simulink model "coefficientOfFriction_2017a_directVcommand"  (R2017a)
settings: Solver=FixedStepDiscrete  StartTime=0.0  StopTime=inf  FixedStep=mdl_T_sample  RelTol=1e-3
undefined symbols (not defined in the file): ctrl_angVel_pid_k_d, ctrl_angVel_pid_k_i, ctrl_angVel_pid_k_p, DiscIntNeverNeededParam, gyro_k_raw2rps, gyro_x_bias, gyro_x_reset, gyro_y_bias, gyro_y_reset, gyro_z_bias, gyro_z_reset, io_read_rateTransition_initialCondition, k_intmax_uint8, mdl, mdl_T_sample, mdl_v_supply, mtr_encoder_countPerRev, mtr_encoder_filter_z_den, mtr_encoder_filter_z_num, mtr_encoder_filter_z_ss_A, mtr_encoder_filter_z_ss_B, mtr_encoder_filter_z_ss_C, mtr_encoder_filter_z_ss_D, mtr_encoder_radPerRev, ui_mtr_w_cmd_dmax, ui_mtr_w_cmd_dmin, ui_mtr_w_cmd_rps, ui_mtr_w_cmd_tStart
libraries: svdutilitieslib x14, simulink x6, arduinolib x5, MinSegLibrary_M2V3 x2, RASPlib x1
settings Model: ExtModeTrigDuration=2  Creator=kando  LastModifiedBy=kando
settings DataIOCC: SaveOutput=off  SignalLogging=off  DSMLogging=off  VisualizeSimOutput=off  SaveTime=off
settings OptimizationCC: LifeSpan=Inf  MaxStackSize=64  SimCompilerOptimization=on  AccelVerboseBuild=on
settings DebuggingCC: AllowSymbolicDim=off  SFUnexpectedBacktrackingDiag=warning  SFNoUnconditionalDefaultTransitionDiag=warning  SFExecutionAtInitializationDiag=none
settings HardwareCC: ProdBitPerInt=16  ProdBitPerPointer=16  ProdBitPerSizeT=16  ProdBitPerPtrDiffT=16  ProdLargestAtomicFloat=None  ProdWordSize=8  ProdHWDeviceType=Atmel->AVR  UseEmbeddedCoderFeatures=off  UseSimulinkCoderFeatures=off
settings ModelReferenceCC: PropagateSignalLabelsOutOfModel=off
settings SFSimCC: MATLABDynamicMemAlloc=off
settings RTWCC: SystemTargetFile=ert.tlc  HardwareBoard=Arduino Mega 2560  TLCOptions=-aInlineSetEventsForThisBaseRateFcn=TLC_FALSE -aSuppressMultiTaskScheduler=TLC_FALSE -aRateBasedStepFcn=1  TemplateMakefile=ert_default_tmf  Description=Embedded Coder  Toolchain=Arduino AVR  BuildConfiguration=Faster Runs
settings ERTTargetCC: MultiwordLength=2048  ERTCustomFileBanners=off  SupportContinuousTime=on  SupportNonInlinedSFcns=on  RemoveResetFunc=off  SupportVariableSizeSignals=on  ModelStepFunctionPrototypeControlCompliant=off  ConvertIfToSwitch=off  SuppressUnreachableDefaultCases=off
settings ConfigComp: CovMetricSettings=dw  CovHtmlReporting=on  CovSaveCumulativeToWorkspaceVar=on  CovSaveSingleToWorkspaceVar=on  CovExternalEMLEnable=off

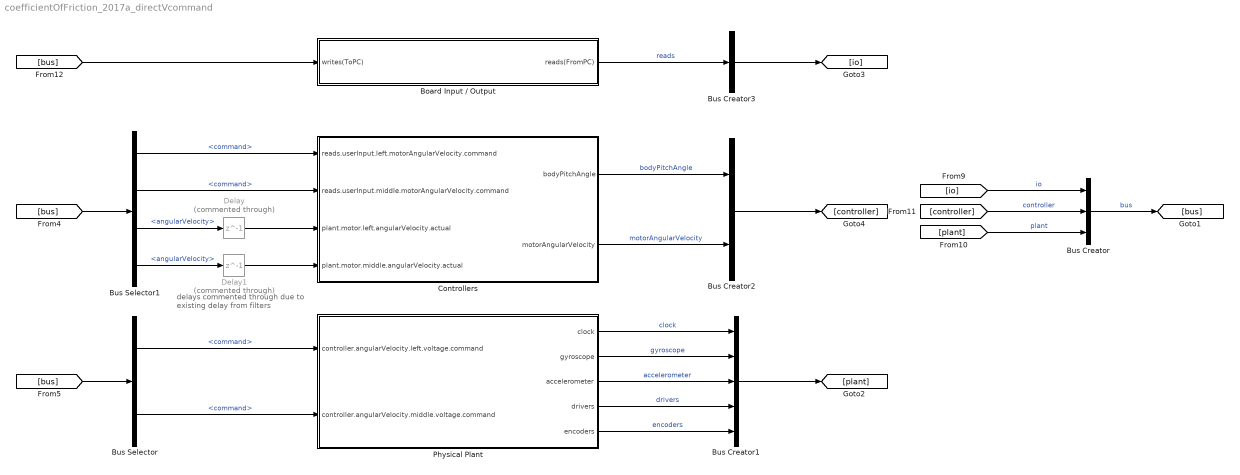
== system coefficientOfFriction_2017a_directVcommand ==
  note: delays commented through
      | due to existing delay from filters
  Board Input / Output : Subsystem
  Bus Creator : BusCreator  Inputs=3
  Bus Creator1 : BusCreator  Inputs=5
  Bus Creator2 : BusCreator  Inputs=2
  Bus Creator3 : BusCreator  Inputs=1
  Bus Selector : BusSelector  OutputSignals=controller.motorAngularVelocity.left.voltage.command,controller.motorAngularVelocity.middle.voltage.command
  Bus Selector1 : BusSelector  OutputSignals=io.reads.userInput.motorAngularVelocity.command,io.reads.userInput.motorAngularVelocity.command,plant.encoders.left.angularVelocity,plant.encoders.middle.angularVelocity
  Controllers : Subsystem
  Delay : Delay  Commented=through  DelayLength=1
  Delay1 : Delay  Commented=through  DelayLength=1
  Physical Plant : Subsystem
  wires:
  Controllers/2(motorAngularVelocity) -> Bus Creator2/2  "motorAngularVelocity"
  Physical Plant/2(gyroscope) -> Bus Creator1/2  "gyroscope"
  Physical Plant/3(accelerometer) -> Bus Creator1/3  "accelerometer"
  Physical Plant/5(encoders) -> Bus Creator1/5  "encoders"
  Bus Creator1/1 -> [plant]
  [io] -> Bus Creator/1  "io"
  [controller] -> Bus Creator/2  "controller"
  [plant] -> Bus Creator/3  "plant"
  Bus Creator/1 -> [bus]  "bus"
  Bus Creator2/1 -> [controller]
  Controllers/1(bodyPitchAngle) -> Bus Creator2/1  "bodyPitchAngle"
  [bus] -> Board Input / Output/1(writes(ToPC))
  Bus Creator3/1 -> [io]
  Board Input / Output/1(reads(FromPC)) -> Bus Creator3/1  "reads"
  [bus] -> Bus Selector1/1
  Bus Selector1/4 -> Delay1/1  "<angularVelocity>"
  Bus Selector1/3 -> Delay/1  "<angularVelocity>"
  Delay/1 -> Controllers/3(plant.motor.left.angularVelocity.actual)
  Delay1/1 -> Controllers/4(plant.motor.middle.angularVelocity.actual)
  Physical Plant/1(clock) -> Bus Creator1/1  "clock"
  Bus Selector/1 -> Physical Plant/1(controller.angularVelocity.left.voltage.command)  "<command>"
  Bus Selector/2 -> Physical Plant/2(controller.angularVelocity.middle.voltage.command)  "<command>"
  [bus] -> Bus Selector/1
  Physical Plant/4(drivers) -> Bus Creator1/4  "drivers"
  Bus Selector1/1 -> Controllers/1("reads.userInput.left.motorAngularVelocity.command ")  "<command>"
  Bus Selector1/2 -> Controllers/2("reads.userInput.middle.motorAngularVelocity.command ")  "<command>"

== system coefficientOfFriction_2017a_directVcommand/Board Input // Output ==
  writes(ToPC) : Inport
  Bus Creator3 : BusCreator  Inputs=1
  Reads (From PC) : Subsystem
  Writes (To PC) : Subsystem  Variant=on  VariantControl=Variant1  OverrideUsingVariant=(default)
  reads(FromPC) : Outport
  wires:
  Reads (From PC)/1(userInput) -> Bus Creator3/1  "userInput"
  Bus Creator3/1 -> reads(FromPC)/1
  writes(ToPC)/1 -> Writes (To PC)/1("systemSignalBus ")

== system coefficientOfFriction_2017a_directVcommand/Controllers ==
  "reads.userInput.left.motorAngularVelocity.command " : Inport
  "reads.userInput.middle.motorAngularVelocity.command " : Inport  Port=2
  plant.motor.left.angularVelocity.actual : Inport  Port=3
  plant.motor.middle.angularVelocity.actual : Inport  Port=4
  Bus Creator : BusCreator  Inputs=2
  Constant : Constant  Value=0  SampleTime=mdl_T_sample
  Motor Angular Velocity : Subsystem  Variant=on  VariantControl=Variant1  OverrideUsingVariant=Variant1
  bodyPitchAngle : Outport
  motorAngularVelocity : Outport  Port=2
  wires:
  Motor Angular Velocity/1(left) -> Bus Creator/1  "left"
  Motor Angular Velocity/2(middle) -> Bus Creator/2  "middle"
  Bus Creator/1 -> motorAngularVelocity/1
  "reads.userInput.left.motorAngularVelocity.command "/1 -> Motor Angular Velocity/1("left.motorAngularVelocity.command ")
  plant.motor.left.angularVelocity.actual/1 -> Motor Angular Velocity/2(left.motorAngularVelocity.measured)
  "reads.userInput.middle.motorAngularVelocity.command "/1 -> Motor Angular Velocity/3("middle.motorAngularVelocity.command ")
  plant.motor.middle.angularVelocity.actual/1 -> Motor Angular Velocity/4(middle.motorAngularVelocity.measured)
  Constant/1 -> bodyPitchAngle/1

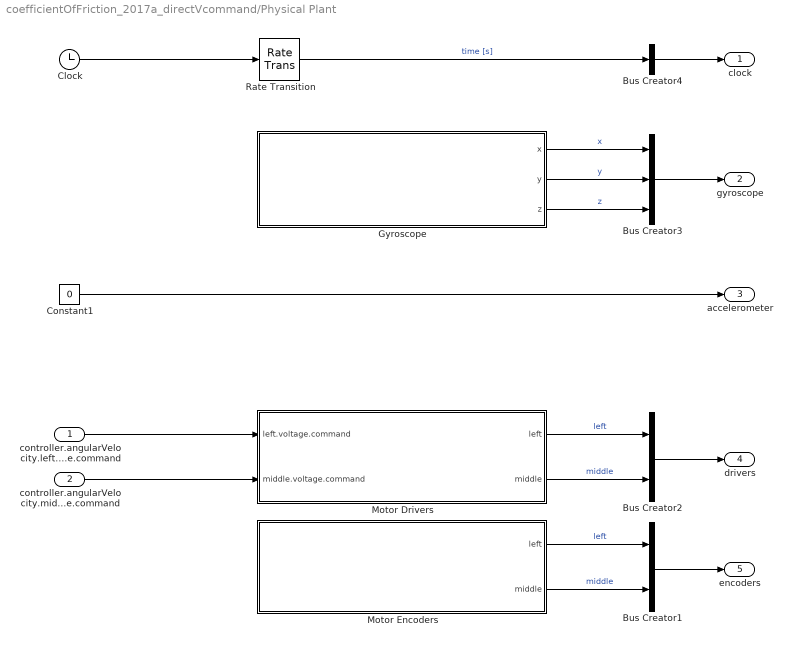
== system coefficientOfFriction_2017a_directVcommand/Physical Plant ==
  controller.angularVelocity.left.voltage.command : Inport
  controller.angularVelocity.middle.voltage.command : Inport  Port=2
  Bus Creator1 : BusCreator  Inputs=2
  Bus Creator2 : BusCreator  Inputs=2
  Bus Creator3 : BusCreator  Inputs=3
  Bus Creator4 : BusCreator  Inputs=1
  Clock : Clock
      settings: Decimation=round( 1 / mdl_T_sample )
  Constant1 : Constant  Value=0  SampleTime=mdl_T_sample
  Gyroscope : Subsystem
  Motor Drivers : Subsystem
  Motor Encoders : Subsystem
  Rate Transition : RateTransition  OutPortSampleTime=mdl_T_sample
  clock : Outport
  gyroscope : Outport  Port=2
  accelerometer : Outport  Port=3
  drivers : Outport  Port=4
  encoders : Outport  Port=5
  wires:
  Clock/1 -> Rate Transition/1
  Motor Encoders/1(left) -> Bus Creator1/1  "left"
  Motor Encoders/2(middle) -> Bus Creator1/2  "middle"
  Constant1/1 -> accelerometer/1
  Motor Drivers/2(middle) -> Bus Creator2/2  "middle"
  Motor Drivers/1(left) -> Bus Creator2/1  "left"
  Bus Creator2/1 -> drivers/1
  Bus Creator1/1 -> encoders/1
  Rate Transition/1 -> Bus Creator4/1  "time [s]"
  Gyroscope/1(x) -> Bus Creator3/1  "x"
  Gyroscope/2(y) -> Bus Creator3/2  "y"
  Gyroscope/3(z) -> Bus Creator3/3  "z"
  Bus Creator3/1 -> gyroscope/1
  controller.angularVelocity.left.voltage.command/1 -> Motor Drivers/1(left.voltage.command)
  controller.angularVelocity.middle.voltage.command/1 -> Motor Drivers/2(middle.voltage.command)
  Bus Creator4/1 -> clock/1

== system coefficientOfFriction_2017a_directVcommand/Board Input // Output/Reads (From PC) ==
  Bus Creator1 : BusCreator  Inputs=1
  Bus Creator3 : BusCreator  Inputs=1
  Data Type Conversion9 : DataTypeConversion  OutDataTypeStr=double
  Gain3 : Gain  Gain=ui_mtr_w_cmd_rps
      settings: AttributesFormatString=%<Gain>
  Rate Limiter : RateLimiter  RisingSlewLimit=ui_mtr_w_cmd_dmax  FallingSlewLimit=ui_mtr_w_cmd_dmin  SampleTimeMode=inherited
  Step : Step  Time=ui_mtr_w_cmd_tStart  SampleTime=mdl_T_sample
  userInput : Outport
  wires:
  Bus Creator3/1 -> userInput/1
  Bus Creator1/1 -> Bus Creator3/1  "motorAngularVelocity"
  Data Type Conversion9/1 -> Bus Creator1/1  "command"
  Gain3/1 -> Data Type Conversion9/1
  Step/1 -> Rate Limiter/1
  Rate Limiter/1 -> Gain3/1

== system coefficientOfFriction_2017a_directVcommand/Board Input // Output/Writes (To PC) ==
  "systemSignalBus " : Inport
  Scopes : Subsystem  VariantControl=Variant1
  Serial : Subsystem  VariantControl=(default)

== system coefficientOfFriction_2017a_directVcommand/Controllers/Motor Angular Velocity ==
  "left.motorAngularVelocity.command " : Inport
  left.motorAngularVelocity.measured : Inport  Port=2
  "middle.motorAngularVelocity.command " : Inport  Port=3
  middle.motorAngularVelocity.measured : Inport  Port=4
  PID : Subsystem  VariantControl=Variant1
  left : Outport
  middle : Outport  Port=2

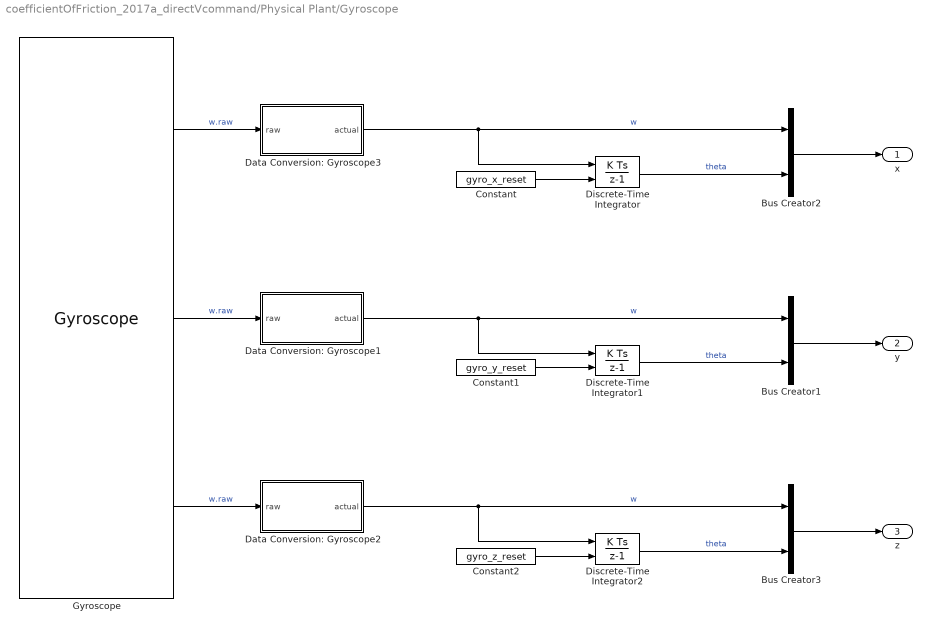
== system coefficientOfFriction_2017a_directVcommand/Physical Plant/Gyroscope ==
  Bus Creator1 : BusCreator  Inputs=2
  Bus Creator2 : BusCreator  Inputs=2
  Bus Creator3 : BusCreator  Inputs=2
  Constant : Constant  Value=gyro_x_reset  SampleTime=mdl_T_sample
  Constant1 : Constant  Value=gyro_y_reset  SampleTime=mdl_T_sample
  Constant2 : Constant  Value=gyro_z_reset  SampleTime=mdl_T_sample
  Data Conversion: Gyroscope1 : Subsystem  mask{gyro_bias=gyro_y_bias}
      mask prompts: gyro_bias "Bias"
      settings: AttributesFormatString=bias: %<gyro_bias>
  Data Conversion: Gyroscope2 : Subsystem  mask{gyro_bias=gyro_z_bias}
      mask prompts: gyro_bias "Bias"
      settings: AttributesFormatString=bias: %<gyro_bias>
  Data Conversion: Gyroscope3 : Subsystem  mask{gyro_bias=gyro_x_bias}
      mask prompts: gyro_bias "Bias"
      settings: AttributesFormatString=bias: %<gyro_bias>
  Discrete-Time Integrator : DiscreteIntegrator  ExternalReset=either  InitialConditionSetting=State (most efficient)  SampleTime=mdl_T_sample  ICPrevOutput=DiscIntNeverNeededParam  ICPrevScaledInput=DiscIntNeverNeededParam
  Discrete-Time Integrator1 : DiscreteIntegrator  ExternalReset=either  InitialConditionSetting=State (most efficient)  SampleTime=mdl_T_sample  ICPrevOutput=DiscIntNeverNeededParam  ICPrevScaledInput=DiscIntNeverNeededParam
  Discrete-Time Integrator2 : DiscreteIntegrator  ExternalReset=either  InitialConditionSetting=State (most efficient)  SampleTime=mdl_T_sample  ICPrevOutput=DiscIntNeverNeededParam  ICPrevScaledInput=DiscIntNeverNeededParam
  Gyroscope : RASPlib/Gyroscope  DLPFmode=gyro_dlpf_mode
      settings: AttributesFormatString=DLPF mode: %<DLPFmode>  SourceProductName=Rensselaer Arduino Support Package
  x : Outport
  y : Outport  Port=2
  z : Outport  Port=3
  wires:
  Gyroscope/2 -> Data Conversion: Gyroscope1/1(raw)  "w.raw"
  Gyroscope/1 -> Data Conversion: Gyroscope3/1(raw)  "w.raw"
  Gyroscope/3 -> Data Conversion: Gyroscope2/1(raw)  "w.raw"
  Data Conversion: Gyroscope3/1(actual) -> Bus Creator2/1, Discrete-Time Integrator/1  "w"
  Constant/1 -> Discrete-Time Integrator/2
  Constant1/1 -> Discrete-Time Integrator1/2
  Constant2/1 -> Discrete-Time Integrator2/2
  Discrete-Time Integrator/1 -> Bus Creator2/2  "theta"
  Discrete-Time Integrator1/1 -> Bus Creator1/2  "theta"
  Data Conversion: Gyroscope1/1(actual) -> Discrete-Time Integrator1/1, Bus Creator1/1  "w"
  Data Conversion: Gyroscope2/1(actual) -> Discrete-Time Integrator2/1, Bus Creator3/1  "w"
  Discrete-Time Integrator2/1 -> Bus Creator3/2  "theta"
  Bus Creator2/1 -> x/1
  Bus Creator1/1 -> y/1
  Bus Creator3/1 -> z/1

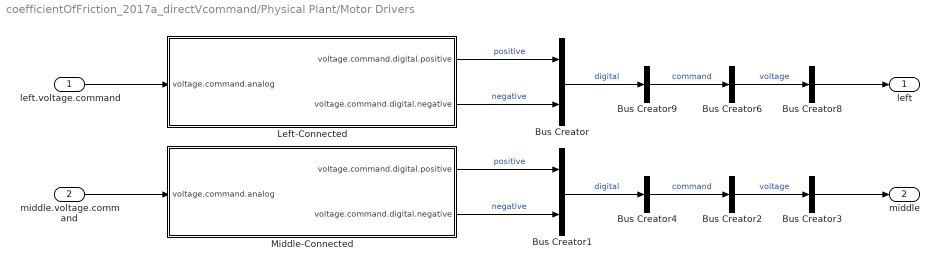
== system coefficientOfFriction_2017a_directVcommand/Physical Plant/Motor Drivers ==
  left.voltage.command : Inport
  middle.voltage.command : Inport  Port=2
  Bus Creator : BusCreator  Inputs=2
  Bus Creator1 : BusCreator  Inputs=2
  Bus Creator{2..4,6,8..9} (6 alike) : BusCreator  Inputs=1
  Left-Connected : Subsystem
  Middle-Connected : Subsystem
  left : Outport
  middle : Outport  Port=2
  wires:
  Bus Creator/1 -> Bus Creator9/1  "digital"
  Left-Connected/1(voltage.command.digital.positive) -> Bus Creator/1  "positive"
  Left-Connected/2(voltage.command.digital.negative) -> Bus Creator/2  "negative"
  Bus Creator6/1 -> Bus Creator8/1  "voltage"
  left.voltage.command/1 -> Left-Connected/1(voltage.command.analog)
  middle.voltage.command/1 -> Middle-Connected/1(voltage.command.analog)
  Bus Creator8/1 -> left/1
  Bus Creator9/1 -> Bus Creator6/1  "command"
  Bus Creator4/1 -> Bus Creator2/1  "command"
  Bus Creator3/1 -> middle/1
  Bus Creator2/1 -> Bus Creator3/1  "voltage"
  Middle-Connected/2(voltage.command.digital.negative) -> Bus Creator1/2  "negative"
  Middle-Connected/1(voltage.command.digital.positive) -> Bus Creator1/1  "positive"
  Bus Creator1/1 -> Bus Creator4/1  "digital"

== system coefficientOfFriction_2017a_directVcommand/Physical Plant/Motor Encoders ==
  Bus Creator : BusCreator  Inputs=2
  Bus Creator1 : BusCreator  Inputs=2
  Left-Connected : Subsystem
  Middle-Connected : Subsystem
  left : Outport
  middle : Outport  Port=2
  wires:
  Bus Creator1/1 -> middle/1
  Bus Creator/1 -> left/1
  Middle-Connected/1(position.measured) -> Bus Creator1/1  "position"
  Middle-Connected/2(angularVelocity.calculated) -> Bus Creator1/2  "angularVelocity"
  Left-Connected/1(position.measured) -> Bus Creator/1  "position"
  Left-Connected/2(angularVelocity.calculated) -> Bus Creator/2  "angularVelocity"

== system coefficientOfFriction_2017a_directVcommand/Board Input // Output/Writes (To PC)/Scopes ==
  systemSignalBus : Inport
  Bus Selector1 : BusSelector  OutputSignals=plant.clock,io.reads.userInput.motorAngularVelocity.command,plant.encoders.left.angularVelocity,controller.motorAngularVelocity.left.angularVelocity.error,controller.motorAngularVelocity.left.voltage.command,io.reads.userInput.motorAngularVelocity.command,plant.encoders.middle.angularVelocity,controller.motorAngularVelocity.middle.angularVelocity.error,controller.motorAngularVelocity.middle.voltage.command,plant.drivers.left.voltage.command.digital,plant.drivers.left.voltage.sign.digital,plant.drivers.middle.voltage.command.digital,plant.drivers.middle.voltage.sign.digital
  Mux : Mux  Commented=on  Inputs=3
  Scope : Scope
  Scope1 : Scope  NumInputPorts=4
  Scope2 : Scope  NumInputPorts=4
  Scope3 : Scope  NumInputPorts=4
  wires:
  Bus Selector1/1 -> Scope/1  "<clock>"
  systemSignalBus/1 -> Bus Selector1/1
  Bus Selector1/2 -> Scope1/1  "<command>"
  Bus Selector1/3 -> Scope1/2  "<angularVelocity>"
  Bus Selector1/4 -> Scope1/3  "<error>"
  Bus Selector1/5 -> Scope1/4  "<command>"
  Bus Selector1/6 -> Scope2/1  "<command>"
  Bus Selector1/7 -> Scope2/2  "<angularVelocity>"
  Bus Selector1/8 -> Scope2/3  "<error>"
  Bus Selector1/9 -> Scope2/4  "<command>"
  Bus Selector1/10 -> Scope3/1  "<digital>"
  Bus Selector1/11 -> Scope3/2  "<digital>"
  Bus Selector1/12 -> Scope3/3  "<digital>"
  Bus Selector1/13 -> Scope3/4  "<digital>"

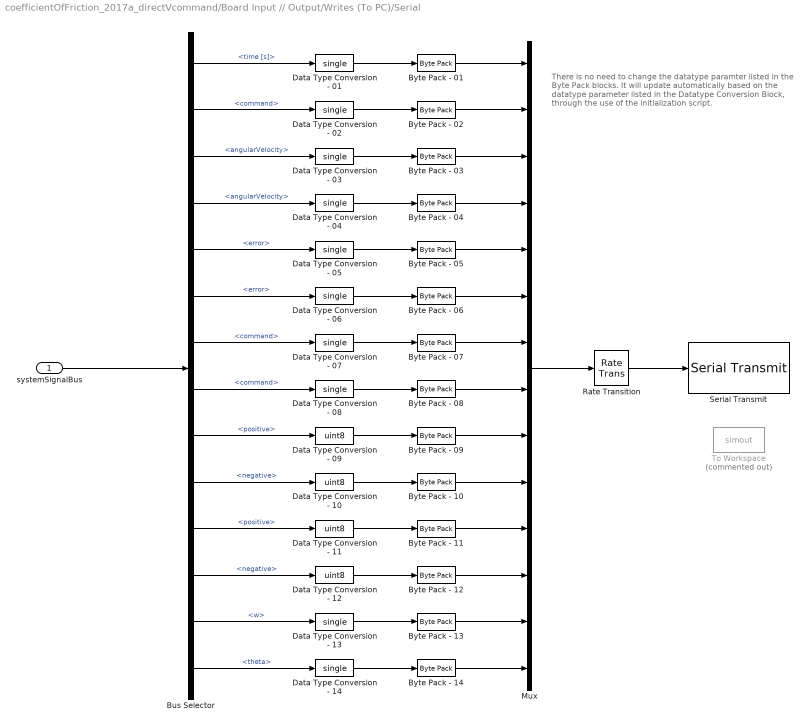
== system coefficientOfFriction_2017a_directVcommand/Board Input // Output/Writes (To PC)/Serial ==
  note: There is no need to change the datatype paramter
      | listed in the Byte Pack blocks.
      |
      | It will update automatically based on the datatype parameter
      | listed in the Datatype Conversion Block,
      | through the use of the initialization script.
  systemSignalBus : Inport
  Bus Selector : BusSelector  OutputSignals=plant.clock.time [s],io.reads.userInput.motorAngularVelocity.command,plant.encoders.left.angularVelocity,plant.encoders.middle.angularVelocity,controller.motorAngularVelocity.left.angularVelocity.error,controller.motorAngularVelocity.middle.angularVelocity.error,controller.motorAngularVelocity.left.voltage.command,controller.motorAngularVelocity.middle.voltage.command,plant.drivers.left.voltage.command.digital.positive,plant.drivers.left.voltage.command.digital.negative,plant.drivers.middle.voltage.command.digital.positive,plant.drivers.middle.voltage.command.digital.negative,plant.gyroscope.x.w,plant.gyroscope.x.theta
  Byte Pack - 01 : svdutilitieslib/Byte Pack  datatypes={'single'}  byteAlign=1  blockPlatform=arduinoert
      settings: AttributesFormatString=%<datatypes>  SourceProductName=Simulink Support Package for Arduino Hardware
  Byte Pack - 02 : svdutilitieslib/Byte Pack  datatypes={'single'}  byteAlign=1  blockPlatform=arduinoert
      settings: AttributesFormatString=%<datatypes>  SourceProductName=Simulink Support Package for Arduino Hardware
  Byte Pack - 03 : svdutilitieslib/Byte Pack  datatypes={'single'}  byteAlign=1  blockPlatform=arduinoert
      settings: AttributesFormatString=%<datatypes>  SourceProductName=Simulink Support Package for Arduino Hardware
  Byte Pack - 04 : svdutilitieslib/Byte Pack  datatypes={'single'}  byteAlign=1  blockPlatform=arduinoert
      settings: AttributesFormatString=%<datatypes>  SourceProductName=Simulink Support Package for Arduino Hardware
  Byte Pack - 05 : svdutilitieslib/Byte Pack  datatypes={'single'}  byteAlign=1  blockPlatform=arduinoert
      settings: AttributesFormatString=%<datatypes>  SourceProductName=Simulink Support Package for Arduino Hardware
  Byte Pack - 06 : svdutilitieslib/Byte Pack  datatypes={'single'}  byteAlign=1  blockPlatform=arduinoert
      settings: AttributesFormatString=%<datatypes>  SourceProductName=Simulink Support Package for Arduino Hardware
  Byte Pack - 07 : svdutilitieslib/Byte Pack  datatypes={'single'}  byteAlign=1  blockPlatform=arduinoert
      settings: AttributesFormatString=%<datatypes>  SourceProductName=Simulink Support Package for Arduino Hardware
  Byte Pack - 08 : svdutilitieslib/Byte Pack  datatypes={'single'}  byteAlign=1  blockPlatform=arduinoert
      settings: AttributesFormatString=%<datatypes>  SourceProductName=Simulink Support Package for Arduino Hardware
  Byte Pack - 09 : svdutilitieslib/Byte Pack  datatypes={'uint8'}  byteAlign=1  blockPlatform=arduinoert
      settings: AttributesFormatString=%<datatypes>  SourceProductName=Simulink Support Package for Arduino Hardware
  Byte Pack - 10 : svdutilitieslib/Byte Pack  datatypes={'uint8'}  byteAlign=1  blockPlatform=arduinoert
      settings: AttributesFormatString=%<datatypes>  SourceProductName=Simulink Support Package for Arduino Hardware
  Byte Pack - 11 : svdutilitieslib/Byte Pack  datatypes={'uint8'}  byteAlign=1  blockPlatform=arduinoert
      settings: AttributesFormatString=%<datatypes>  SourceProductName=Simulink Support Package for Arduino Hardware
  Byte Pack - 12 : svdutilitieslib/Byte Pack  datatypes={'uint8'}  byteAlign=1  blockPlatform=arduinoert
      settings: AttributesFormatString=%<datatypes>  SourceProductName=Simulink Support Package for Arduino Hardware
  Byte Pack - 13 : svdutilitieslib/Byte Pack  datatypes={'single'}  byteAlign=1  blockPlatform=arduinoert
      settings: AttributesFormatString=%<datatypes>  SourceProductName=Simulink Support Package for Arduino Hardware
  Byte Pack - 14 : svdutilitieslib/Byte Pack  datatypes={'single'}  byteAlign=1  blockPlatform=arduinoert
      settings: AttributesFormatString=%<datatypes>  SourceProductName=Simulink Support Package for Arduino Hardware
  Data Type Conversion - 01 : DataTypeConversion  OutDataTypeStr=single
  Data Type Conversion - 02 : DataTypeConversion  OutDataTypeStr=single
  Data Type Conversion - 03 : DataTypeConversion  OutDataTypeStr=single
  Data Type Conversion - 04 : DataTypeConversion  OutDataTypeStr=single
  Data Type Conversion - 05 : DataTypeConversion  OutDataTypeStr=single
  Data Type Conversion - 06 : DataTypeConversion  OutDataTypeStr=single
  Data Type Conversion - 07 : DataTypeConversion  OutDataTypeStr=single
  Data Type Conversion - 08 : DataTypeConversion  OutDataTypeStr=single
  Data Type Conversion - 09 : DataTypeConversion  OutDataTypeStr=uint8
  Data Type Conversion - 10 : DataTypeConversion  OutDataTypeStr=uint8
  Data Type Conversion - 11 : DataTypeConversion  OutDataTypeStr=uint8
  Data Type Conversion - 12 : DataTypeConversion  OutDataTypeStr=uint8
  Data Type Conversion - 13 : DataTypeConversion  OutDataTypeStr=single
  Data Type Conversion - 14 : DataTypeConversion  OutDataTypeStr=single
  Mux : Mux  Inputs=14
  Rate Transition : RateTransition  X0=io_read_rateTransition_initialCondition  OutPortSampleTimeMultiple=io_read_rateTransition_decimation  OutPortSampleTime=io_read_rateTransition_T_sample
  Serial Transmit : arduinolib/Serial Transmit  portNumber=0  sendmode=write  sendformat=Decimal  floatprecision=2  blockPlatform=arduino
      settings: SourceProductName=Simulink Support Package for Arduino Hardware
  To Workspace : ToWorkspace  Commented=on  VariableName=simout  SaveFormat=Timeseries  SampleTime=-1
  wires:
  Byte Pack - 04/1 -> Mux/4
  Byte Pack - 03/1 -> Mux/3
  Byte Pack - 07/1 -> Mux/7
  Mux/1 -> Rate Transition/1
  Byte Pack - 01/1 -> Mux/1
  Byte Pack - 06/1 -> Mux/6
  Byte Pack - 05/1 -> Mux/5
  Byte Pack - 08/1 -> Mux/8
  Byte Pack - 02/1 -> Mux/2
  systemSignalBus/1 -> Bus Selector/1
  Bus Selector/2 -> Data Type Conversion - 02/1  "<command>"
  Bus Selector/9 -> Data Type Conversion - 09/1  "<positive>"
  Bus Selector/10 -> Data Type Conversion - 10/1  "<negative>"
  Byte Pack - 09/1 -> Mux/9
  Byte Pack - 10/1 -> Mux/10
  Data Type Conversion - 01/1 -> Byte Pack - 01/1
  Data Type Conversion - 02/1 -> Byte Pack - 02/1
  Data Type Conversion - 03/1 -> Byte Pack - 03/1
  Data Type Conversion - 04/1 -> Byte Pack - 04/1
  Data Type Conversion - 05/1 -> Byte Pack - 05/1
  Data Type Conversion - 06/1 -> Byte Pack - 06/1
  Data Type Conversion - 07/1 -> Byte Pack - 07/1
  Data Type Conversion - 08/1 -> Byte Pack - 08/1
  Data Type Conversion - 09/1 -> Byte Pack - 09/1
  Data Type Conversion - 10/1 -> Byte Pack - 10/1
  Data Type Conversion - 12/1 -> Byte Pack - 12/1
  Data Type Conversion - 11/1 -> Byte Pack - 11/1
  Bus Selector/12 -> Data Type Conversion - 12/1  "<negative>"
  Bus Selector/11 -> Data Type Conversion - 11/1  "<positive>"
  Byte Pack - 11/1 -> Mux/11
  Byte Pack - 12/1 -> Mux/12
  Bus Selector/3 -> Data Type Conversion - 03/1  "<angularVelocity>"
  Bus Selector/4 -> Data Type Conversion - 04/1  "<angularVelocity>"
  Bus Selector/5 -> Data Type Conversion - 05/1  "<error>"
  Bus Selector/6 -> Data Type Conversion - 06/1  "<error>"
  Bus Selector/7 -> Data Type Conversion - 07/1  "<command>"
  Bus Selector/8 -> Data Type Conversion - 08/1  "<command>"
  Rate Transition/1 -> Serial Transmit/1
  Byte Pack - 13/1 -> Mux/13
  Data Type Conversion - 13/1 -> Byte Pack - 13/1
  Bus Selector/13 -> Data Type Conversion - 13/1  "<w>"
  Data Type Conversion - 14/1 -> Byte Pack - 14/1
  Bus Selector/14 -> Data Type Conversion - 14/1  "<theta>"
  Byte Pack - 14/1 -> Mux/14
  Bus Selector/1 -> Data Type Conversion - 01/1  "<time [s]>"

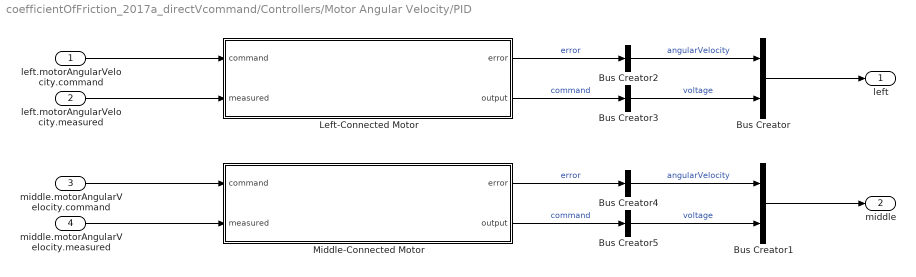
== system coefficientOfFriction_2017a_directVcommand/Controllers/Motor Angular Velocity/PID ==
  "left.motorAngularVelocity.command " : Inport
  left.motorAngularVelocity.measured : Inport  Port=2
  "middle.motorAngularVelocity.command " : Inport  Port=3
  middle.motorAngularVelocity.measured : Inport  Port=4
  Bus Creator : BusCreator  Inputs=2
  Bus Creator1 : BusCreator  Inputs=2
  Bus Creator{2..5} (4 alike) : BusCreator  Inputs=1
  Left-Connected Motor : Subsystem
  Middle-Connected Motor : Subsystem
  left : Outport
  middle : Outport  Port=2
  wires:
  "left.motorAngularVelocity.command "/1 -> Left-Connected Motor/1(command)
  left.motorAngularVelocity.measured/1 -> Left-Connected Motor/2(measured)
  "middle.motorAngularVelocity.command "/1 -> Middle-Connected Motor/1(command)
  middle.motorAngularVelocity.measured/1 -> Middle-Connected Motor/2(measured)
  Left-Connected Motor/2(output) -> Bus Creator3/1  "command"
  Left-Connected Motor/1(error) -> Bus Creator2/1  "error"
  Bus Creator2/1 -> Bus Creator/1  "angularVelocity"
  Bus Creator3/1 -> Bus Creator/2  "voltage"
  Bus Creator/1 -> left/1
  Bus Creator1/1 -> middle/1
  Bus Creator5/1 -> Bus Creator1/2  "voltage"
  Bus Creator4/1 -> Bus Creator1/1  "angularVelocity"
  Middle-Connected Motor/1(error) -> Bus Creator4/1  "error"
  Middle-Connected Motor/2(output) -> Bus Creator5/1  "command"

== system coefficientOfFriction_2017a_directVcommand/Physical Plant/Gyroscope/Data Conversion: Gyroscope1 ==
  raw : Inport
  Add : Sum  Inputs=+-
  Constant : Constant  Value=gyro_bias  SampleTime=mdl_T_sample
  Data Type Conversion1 : DataTypeConversion  OutDataTypeStr=double
  Gain : Gain  Gain=gyro_k_raw2rps
      settings: AttributesFormatString=%<Gain>
  actual : Outport
  wires:
  Gain/1 -> actual/1
  Data Type Conversion1/1 -> Add/1
  raw/1 -> Data Type Conversion1/1
  Constant/1 -> Add/2
  Add/1 -> Gain/1

== system coefficientOfFriction_2017a_directVcommand/Physical Plant/Gyroscope/Data Conversion: Gyroscope2 ==
  raw : Inport
  Add : Sum  Inputs=+-
  Constant : Constant  Value=gyro_bias  SampleTime=mdl_T_sample
  Data Type Conversion1 : DataTypeConversion  OutDataTypeStr=double
  Gain : Gain  Gain=gyro_k_raw2rps
      settings: AttributesFormatString=%<Gain>
  actual : Outport
  wires:
  Add/1 -> Gain/1
  Constant/1 -> Add/2
  raw/1 -> Data Type Conversion1/1
  Data Type Conversion1/1 -> Add/1
  Gain/1 -> actual/1

== system coefficientOfFriction_2017a_directVcommand/Physical Plant/Gyroscope/Data Conversion: Gyroscope3 ==
  raw : Inport
  Add : Sum  Inputs=+-
  Constant : Constant  Value=gyro_bias  SampleTime=mdl_T_sample
  Data Type Conversion1 : DataTypeConversion  OutDataTypeStr=double
  Gain : Gain  Gain=gyro_k_raw2rps
      settings: AttributesFormatString=%<Gain>
  actual : Outport
  wires:
  Add/1 -> Gain/1
  Constant/1 -> Add/2
  raw/1 -> Data Type Conversion1/1
  Data Type Conversion1/1 -> Add/1
  Gain/1 -> actual/1

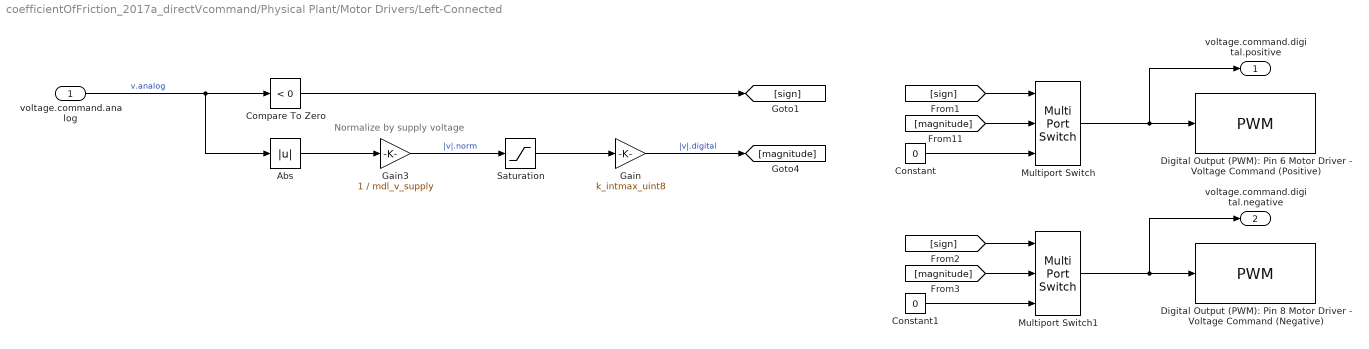
== system coefficientOfFriction_2017a_directVcommand/Physical Plant/Motor Drivers/Left-Connected ==
  note: Normalize by supply voltage
  voltage.command.analog : Inport
  Abs : Abs
  Compare To Zero : simulink/Logic and Bit Operations/Compare To Zero  relop=<  OutDataTypeStr=boolean
  Constant : Constant  Value=0  SampleTime=mdl_T_sample
  Constant1 : Constant  Value=0  OutDataTypeStr=uint8  SampleTime=mdl_T_sample
  Digital Output (PWM): Pin 6 Motor Driver - Voltage Command (Positive) : arduinolib/PWM  pinNumber=6  blockPlatform=arduino
  Digital Output (PWM): Pin 8 Motor Driver - Voltage Command (Negative) : arduinolib/PWM  pinNumber=8  blockPlatform=arduino
  Gain : Gain  Gain=k_intmax_uint8  RndMeth=Round
      settings: AttributesFormatString=%<Gain>
  Gain3 : Gain  Gain=1 / mdl_v_supply
      settings: AttributesFormatString=%<Gain>
  Multiport Switch : MultiPortSwitch  DataPortOrder=Zero-based contiguous  Inputs=2
  Multiport Switch1 : MultiPortSwitch  DataPortOrder=Specify indices  Inputs=2  DataPortIndices={1,0}
  Saturation : Saturate  UpperLimit=+1  LowerLimit=-1
  voltage.command.digital.positive : Outport
  voltage.command.digital.negative : Outport  Port=2
  wires:
  voltage.command.analog/1 -> Abs/1, Compare To Zero/1  "v.analog"
  Gain3/1 -> Saturation/1  "|v|.norm"
  Compare To Zero/1 -> [sign]
  Saturation/1 -> Gain/1
  Gain/1 -> [magnitude]  "|v|.digital"
  [magnitude] -> Multiport Switch/2
  [sign] -> Multiport Switch/1
  Constant/1 -> Multiport Switch/3
  Multiport Switch/1 -> voltage.command.digital.positive/1, Digital Output (PWM): Pin 6 Motor Driver - Voltage Command (Positive)/1
  Multiport Switch1/1 -> voltage.command.digital.negative/1, Digital Output (PWM): Pin 8 Motor Driver - Voltage Command (Negative)/1
  Constant1/1 -> Multiport Switch1/3
  [sign] -> Multiport Switch1/1
  [magnitude] -> Multiport Switch1/2
  Abs/1 -> Gain3/1

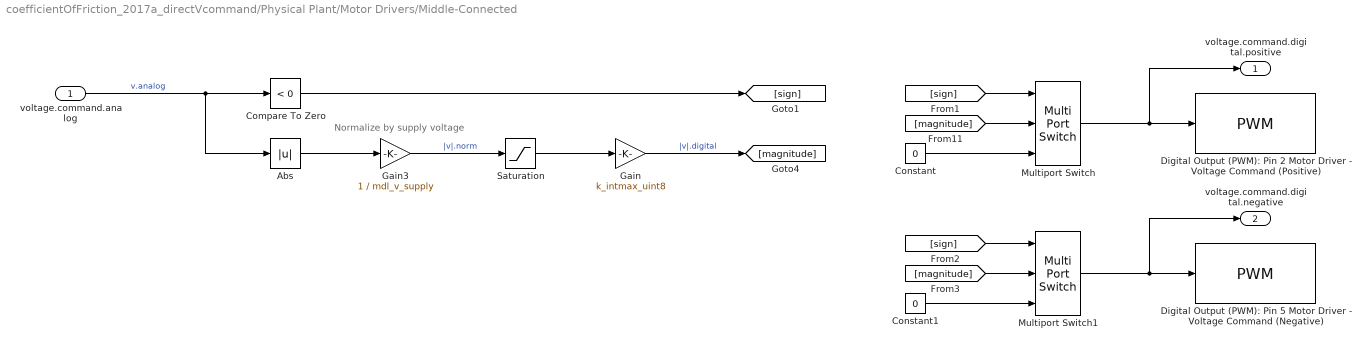
== system coefficientOfFriction_2017a_directVcommand/Physical Plant/Motor Drivers/Middle-Connected ==
  note: Normalize by supply voltage
  voltage.command.analog : Inport
  Abs : Abs
  Compare To Zero : simulink/Logic and Bit Operations/Compare To Zero  relop=<  OutDataTypeStr=boolean
  Constant : Constant  Value=0  SampleTime=mdl_T_sample
  Constant1 : Constant  Value=0  OutDataTypeStr=uint8  SampleTime=mdl_T_sample
  Digital Output (PWM): Pin 2 Motor Driver - Voltage Command (Positive) : arduinolib/PWM  pinNumber=2  blockPlatform=arduino
  Digital Output (PWM): Pin 5 Motor Driver - Voltage Command (Negative) : arduinolib/PWM  pinNumber=5  blockPlatform=arduino
  Gain : Gain  Gain=k_intmax_uint8  RndMeth=Round
      settings: AttributesFormatString=%<Gain>
  Gain3 : Gain  Gain=1 / mdl_v_supply
      settings: AttributesFormatString=%<Gain>
  Multiport Switch : MultiPortSwitch  DataPortOrder=Zero-based contiguous  Inputs=2
  Multiport Switch1 : MultiPortSwitch  DataPortOrder=Specify indices  Inputs=2  DataPortIndices={1,0}
  Saturation : Saturate  UpperLimit=+1  LowerLimit=-1
  voltage.command.digital.positive : Outport
  voltage.command.digital.negative : Outport  Port=2
  wires:
  Abs/1 -> Gain3/1
  [magnitude] -> Multiport Switch1/2
  [sign] -> Multiport Switch1/1
  Constant1/1 -> Multiport Switch1/3
  Multiport Switch1/1 -> Digital Output (PWM): Pin 5 Motor Driver - Voltage Command (Negative)/1, voltage.command.digital.negative/1
  Multiport Switch/1 -> Digital Output (PWM): Pin 2 Motor Driver - Voltage Command (Positive)/1, voltage.command.digital.positive/1
  Constant/1 -> Multiport Switch/3
  [sign] -> Multiport Switch/1
  [magnitude] -> Multiport Switch/2
  Gain/1 -> [magnitude]  "|v|.digital"
  Saturation/1 -> Gain/1
  Compare To Zero/1 -> [sign]
  Gain3/1 -> Saturation/1  "|v|.norm"
  voltage.command.analog/1 -> Compare To Zero/1, Abs/1  "v.analog"

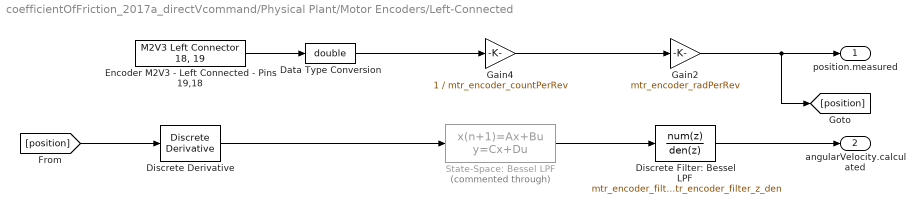
== system coefficientOfFriction_2017a_directVcommand/Physical Plant/Motor Encoders/Left-Connected ==
  Data Type Conversion : DataTypeConversion  OutDataTypeStr=double
      settings: AttributesFormatString=saturateOverflow(%<SaturateOnIntegerOverflow>)
  Discrete Derivative : simulink/Discrete/Discrete Derivative  gainval=1.0  ICPrevScaledInput=0  OutMin=[]  OutMax=[]  OutDataType=fixdt(1, 16)  OutScaling=2^-10  DoSatur=off
      settings: AttributesFormatString=initialCondition = %<ICPrevScaledInput>
  Discrete Filter: Bessel LPF : DiscreteFilter  Numerator=mtr_encoder_filter_z_num  Denominator=mtr_encoder_filter_z_den  SampleTime=mdl_T_sample
      settings: AttributesFormatString=|
      | Num: %<Numerator>
      | Den: %<Denominator>
  Encoder M2V3 - Left Connected - Pins 19,18 : MinSegLibrary_M2V3/M2V3 Left Connector 18, 19  Encoder=1  PinA=19  PinB=18  PWMFSelect=3  PWMTimer=-1
      settings: SourceProductName=Rensselaer Arduino Support Package
  Gain2 : Gain  Gain=mtr_encoder_radPerRev
      settings: AttributesFormatString=%<Gain>
  Gain4 : Gain  Gain=1 / mtr_encoder_countPerRev
      settings: AttributesFormatString=%<Gain>
  State-Space: Bessel LPF : DiscreteStateSpace  Commented=through  A=mtr_encoder_filter_z_ss_A  B=mtr_encoder_filter_z_ss_B  C=mtr_encoder_filter_z_ss_C  D=mtr_encoder_filter_z_ss_D  X0=[0 0]  SampleTime=mdl_T_sample
      settings: AttributesFormatString=|
      | A: %<A>
      | B: %<B>
      | C: %<C>
      | D: %<D>
  position.measured : Outport
  angularVelocity.calculated : Outport  Port=2
  wires:
  Gain4/1 -> Gain2/1
  Discrete Derivative/1 -> State-Space: Bessel LPF/1
  Gain2/1 -> position.measured/1, [position]
  [position] -> Discrete Derivative/1
  Encoder M2V3 - Left Connected - Pins 19,18/1 -> Data Type Conversion/1
  Data Type Conversion/1 -> Gain4/1
  State-Space: Bessel LPF/1 -> Discrete Filter: Bessel LPF/1
  Discrete Filter: Bessel LPF/1 -> angularVelocity.calculated/1

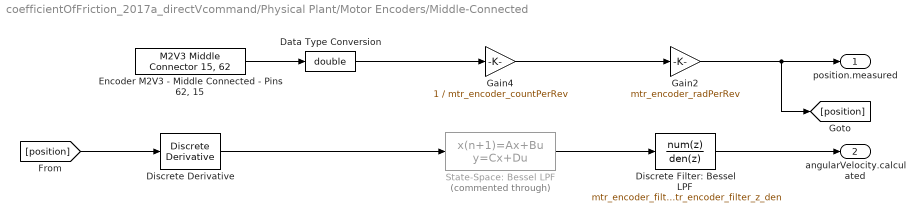
== system coefficientOfFriction_2017a_directVcommand/Physical Plant/Motor Encoders/Middle-Connected ==
  Data Type Conversion : DataTypeConversion  OutDataTypeStr=double
      settings: AttributesFormatString=saturateOverflow(%<SaturateOnIntegerOverflow>)
  Discrete Derivative : simulink/Discrete/Discrete Derivative  gainval=1.0  ICPrevScaledInput=0  OutMin=[]  OutMax=[]  OutDataType=fixdt(1, 16)  OutScaling=2^-10  DoSatur=off
      settings: AttributesFormatString=initialCondition = %<ICPrevScaledInput>
  Discrete Filter: Bessel LPF : DiscreteFilter  Numerator=mtr_encoder_filter_z_num  Denominator=mtr_encoder_filter_z_den  SampleTime=mdl_T_sample
      settings: AttributesFormatString=|
      | Num: %<Numerator>
      | Den: %<Denominator>
  "Encoder M2V3 - Middle Connected - Pins 62, 15" : MinSegLibrary_M2V3/M2V3 Middle Connector 15, 62  Encoder=3  PinA=15  PinB=62  PWMFSelect=3  PWMTimer=-1
      settings: SourceProductName=Rensselaer Arduino Support Package
  Gain2 : Gain  Gain=mtr_encoder_radPerRev
      settings: AttributesFormatString=%<Gain>
  Gain4 : Gain  Gain=1 / mtr_encoder_countPerRev
      settings: AttributesFormatString=%<Gain>
  State-Space: Bessel LPF : DiscreteStateSpace  Commented=through  A=mtr_encoder_filter_z_ss_A  B=mtr_encoder_filter_z_ss_B  C=mtr_encoder_filter_z_ss_C  D=mtr_encoder_filter_z_ss_D  X0=[0 0]  SampleTime=mdl_T_sample
      settings: AttributesFormatString=|
      | A: %<A>
      | B: %<B>
      | C: %<C>
      | D: %<D>
  position.measured : Outport
  angularVelocity.calculated : Outport  Port=2
  wires:
  Data Type Conversion/1 -> Gain4/1
  "Encoder M2V3 - Middle Connected - Pins 62, 15"/1 -> Data Type Conversion/1
  [position] -> Discrete Derivative/1
  Gain2/1 -> [position], position.measured/1
  Gain4/1 -> Gain2/1
  Discrete Filter: Bessel LPF/1 -> angularVelocity.calculated/1
  Discrete Derivative/1 -> State-Space: Bessel LPF/1
  State-Space: Bessel LPF/1 -> Discrete Filter: Bessel LPF/1

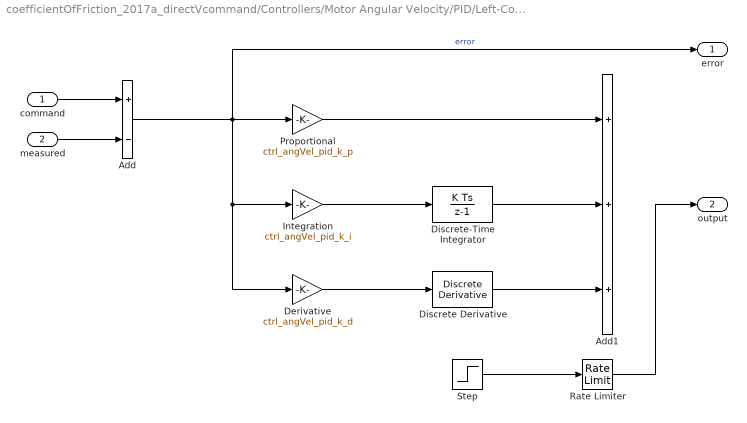
== system coefficientOfFriction_2017a_directVcommand/Controllers/Motor Angular Velocity/PID/Left-Connected Motor ==
  command : Inport
  measured : Inport  Port=2
  Add : Sum  Inputs=+-
  Add1 : Sum  Inputs=+++
  Derivative : Gain  Gain=ctrl_angVel_pid_k_d
      settings: AttributesFormatString=%<Gain>
  Discrete Derivative : simulink/Discrete/Discrete Derivative  gainval=1.0  ICPrevScaledInput=0  OutMin=[]  OutMax=[]  OutDataType=fixdt(1, 16)  OutScaling=2^-10  DoSatur=off
      settings: AttributesFormatString=initialCondition = %<ICPrevScaledInput>
  Discrete-Time Integrator : DiscreteIntegrator  InitialConditionSetting=State (most efficient)  SampleTime=-1  LimitOutput=on  UpperSaturationLimit=+mdl.v.supply  LowerSaturationLimit=-mdl.v.supply  ICPrevOutput=DiscIntNeverNeededParam  ICPrevScaledInput=DiscIntNeverNeededParam
      settings: AttributesFormatString=initialCondition = %<InitialCondition>
  Integration : Gain  Gain=ctrl_angVel_pid_k_i
      settings: AttributesFormatString=%<Gain>
  Proportional : Gain  Gain=ctrl_angVel_pid_k_p
      settings: AttributesFormatString=%<Gain>
  Rate Limiter : RateLimiter  RisingSlewLimit=+0.1  FallingSlewLimit=-0.1  SampleTimeMode=inherited
  Step : Step  Time=0  After=10  SampleTime=mdl_T_sample
  error : Outport
  output : Outport  Port=2
  wires:
  Proportional/1 -> Add1/1
  Add/1 -> error/1, Derivative/1, Integration/1, Proportional/1  "error"
  measured/1 -> Add/2
  command/1 -> Add/1
  Integration/1 -> Discrete-Time Integrator/1
  Derivative/1 -> Discrete Derivative/1
  Discrete-Time Integrator/1 -> Add1/2
  Discrete Derivative/1 -> Add1/3
  Rate Limiter/1 -> output/1
  Step/1 -> Rate Limiter/1

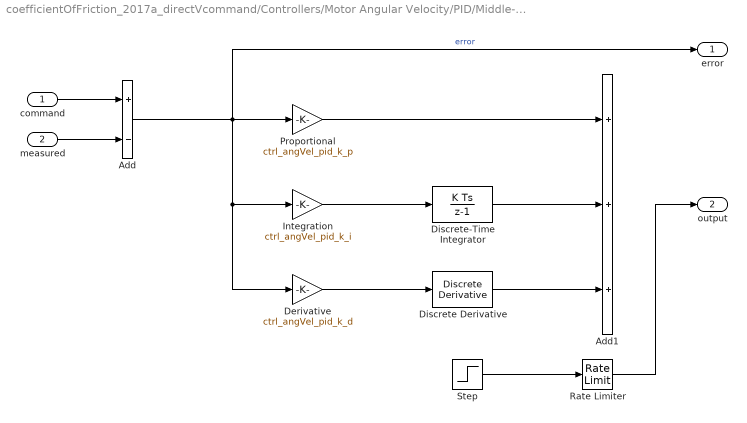
== system coefficientOfFriction_2017a_directVcommand/Controllers/Motor Angular Velocity/PID/Middle-Connected Motor ==
  command : Inport
  measured : Inport  Port=2
  Add : Sum  Inputs=+-
  Add1 : Sum  Inputs=+++
  Derivative : Gain  Gain=ctrl_angVel_pid_k_d
      settings: AttributesFormatString=%<Gain>
  Discrete Derivative : simulink/Discrete/Discrete Derivative  gainval=1.0  ICPrevScaledInput=0  OutMin=[]  OutMax=[]  OutDataType=fixdt(1, 16)  OutScaling=2^-10  DoSatur=off
      settings: AttributesFormatString=initialCondition = %<ICPrevScaledInput>
  Discrete-Time Integrator : DiscreteIntegrator  InitialConditionSetting=State (most efficient)  SampleTime=-1  LimitOutput=on  UpperSaturationLimit=+mdl.v.supply  LowerSaturationLimit=-mdl.v.supply  ICPrevOutput=DiscIntNeverNeededParam  ICPrevScaledInput=DiscIntNeverNeededParam
      settings: AttributesFormatString=initialCondition = %<InitialCondition>
  Integration : Gain  Gain=ctrl_angVel_pid_k_i
      settings: AttributesFormatString=%<Gain>
  Proportional : Gain  Gain=ctrl_angVel_pid_k_p
      settings: AttributesFormatString=%<Gain>
  Rate Limiter : RateLimiter  RisingSlewLimit=+0.1  FallingSlewLimit=-0.1  SampleTimeMode=inherited
  Step : Step  Time=0  After=10  SampleTime=mdl_T_sample
  error : Outport
  output : Outport  Port=2
  wires:
  Discrete Derivative/1 -> Add1/3
  Discrete-Time Integrator/1 -> Add1/2
  Derivative/1 -> Discrete Derivative/1
  Integration/1 -> Discrete-Time Integrator/1
  command/1 -> Add/1
  measured/1 -> Add/2
  Add/1 -> Proportional/1, Integration/1, Derivative/1, error/1  "error"
  Proportional/1 -> Add1/1
  Rate Limiter/1 -> output/1
  Step/1 -> Rate Limiter/1
